simulink model "Simulink7"  (Simulink 5.0)
settings: Solver=FixedStepDiscrete  StartTime=0.0  StopTime=1000.0  FixedStep=1  RelTol=1e-3
undefined symbols (not defined in the file): j, magnitude
libraries: simulink x1
settings Model: Creator=asteele  LastModifiedBy=stevel  ExtModeAutoUpdateStatusClock=off  BooleanDataType=off

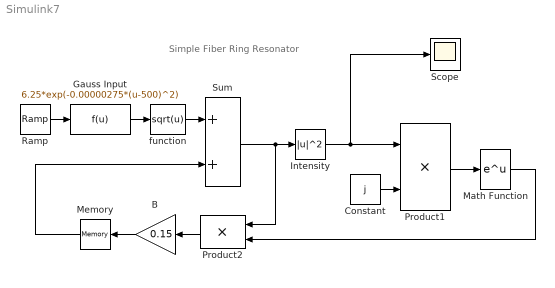
== system Simulink7 ==
  note: Simple Fiber Ring Resonator
  B : Gain  Orientation=left  Gain=0.15  SaturateOnIntegerOverflow=on
  Constant : Constant  Value=j
  Gauss Input : Fcn  Expr=6.25*exp(-0.00000275*(u-500)^2)
  Intensity : Math  Operator=magnitude^2
  Math Function : Math
  Memory : Memory  Orientation=left
  Product1 : Product  SaturateOnIntegerOverflow=on  InputSameDT=on
  Product2 : Product  Orientation=left  SaturateOnIntegerOverflow=on  InputSameDT=on
  Ramp : simulink/Sources/Ramp  slope=1  start=0  X0=0
  Scope : Scope
  Sum : Sum  SaturateOnIntegerOverflow=on  InputSameDT=on
  function : Fcn  Expr=sqrt(u)
  wires:
  Sum/1 -> Intensity/1, Product2/1
  Intensity/1 -> Product1/1, Scope/1
  Product2/1 -> B/1
  B/1 -> Memory/1
  Math Function/1 -> Product2/2
  Constant/1 -> Product1/2
  Product1/1 -> Math Function/1
  Memory/1 -> Sum/2
  Ramp/1 -> Gauss Input/1
  Gauss Input/1 -> function/1
  function/1 -> Sum/1
